simulink model "BatteryModel_Harness"  (R2025b)
settings: Solver=FixedStepDiscrete  StartTime=0.0  StopTime=3600  RelTol=1e-3
libraries: SignalEditorBlockLib x1
settings Model: Creator=sudhakars2  LastModifiedBy=mgmsu

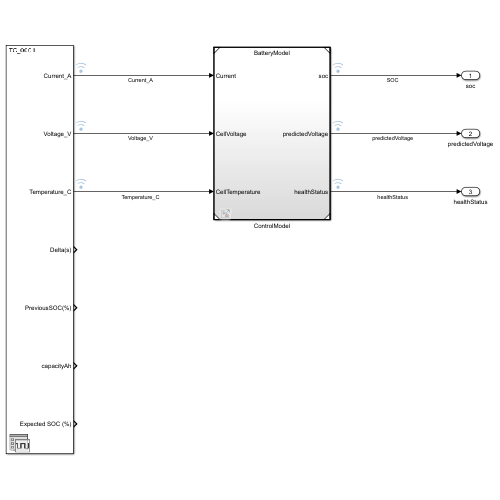
[thumbnail: Simulink's stored preview of the top-level diagram]
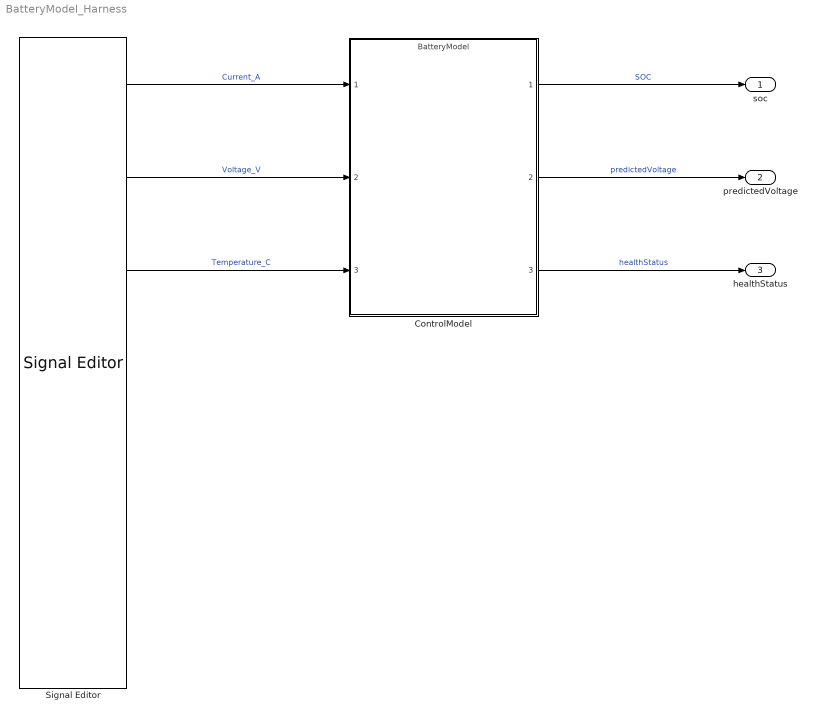
== system BatteryModel_Harness ==
  ControlModel : ModelReference  ModelNameDialog=BatteryModel.slx  SimulationMode=Normal  ModelReferenceVersion=1.25
  Signal Editor : SignalEditorBlockLib/Signal Editor  FileName=TC.mat  ActiveScenario=TC_0001  ActiveSignal=Current_A  IsBus=off  OutputBusObjectStr=Bus: BusObject  SampleTime=0  ZeroCross=off  OutputAfterFinalValue=Setting to zero  Unit=inherit  PreserveSignalName=on  ApplySigPropsToAllScenarios=on  ApplySigPropsToAllSignals=on  SignalPropertySource=Dialog parameters
  soc : Outport
  predictedVoltage : Outport  Port=2
  healthStatus : Outport  Port=3
  wires:
  Signal Editor/1 -> ControlModel/1  "Current_A"
  Signal Editor/2 -> ControlModel/2  "Voltage_V"
  Signal Editor/3 -> ControlModel/3  "Temperature_C"
  ControlModel/1 -> soc/1  "SOC"
  ControlModel/2 -> predictedVoltage/1  "predictedVoltage"
  ControlModel/3 -> healthStatus/1  "healthStatus"
